simulink model "fault_solution_mod"  (R2018b)
settings: Solver=VariableStepAuto  StartTime=0.0  StopTime=10  RelTol=1e-3
values from neighbouring files (symbols this model uses):
  E = [1;1;0;0]    [fault.m]
  F = A1 - K1*C    [fault.m]
  Fx = [1;1;1;1]    [fault.m]
  Fy = [1;1]    [fault.m]
  H = E/((C*E)'*(C*E)) * (C*E)'    [fault.m]
  K = K1 + F*H    [fault.m]
  TB = T*B    [fault.m]
undefined symbols (not defined in the file or in its folder): A, B, C
settings Model: Creator=jal  LastModifiedBy=Ion Sircu

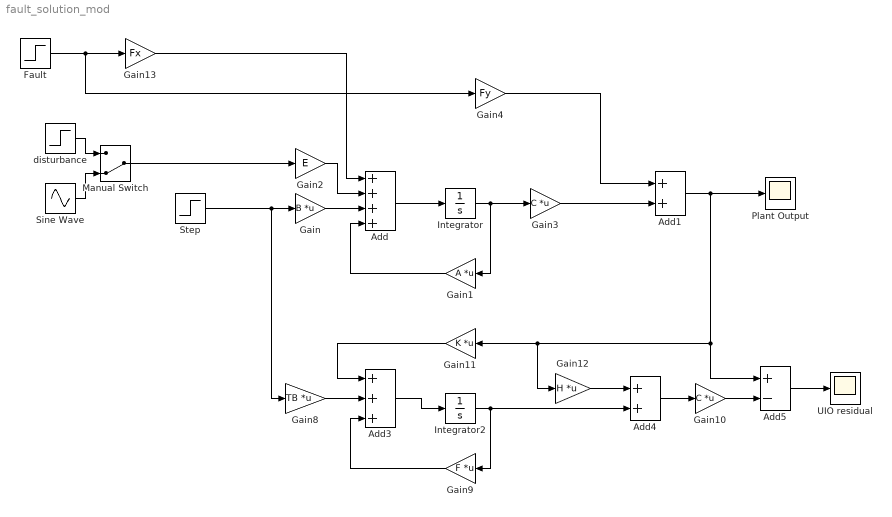
== system fault_solution_mod ==
  Add : Sum  Inputs=++++
  Add1 : Sum
  Add3 : Sum  Inputs=+++
  Add4 : Sum
  Add5 : Sum  Inputs=+-
  Fault : Step  Time=5  After=10  SampleTime=0
  Gain : Gain  Gain=B  Multiplication=Matrix(K*u)
  Gain1 : Gain  Gain=A  Multiplication=Matrix(K*u)
  Gain10 : Gain  Gain=C  Multiplication=Matrix(K*u)
  Gain11 : Gain  Gain=K  Multiplication=Matrix(K*u)
  Gain12 : Gain  Gain=H  Multiplication=Matrix(K*u)
  Gain13 : Gain  Gain=Fx
  Gain2 : Gain  Gain=E
  Gain3 : Gain  Gain=C  Multiplication=Matrix(K*u)
  Gain4 : Gain  Gain=Fy
  Gain8 : Gain  Gain=TB  Multiplication=Matrix(K*u)
  Gain9 : Gain  Gain=F  Multiplication=Matrix(K*u)
  Integrator : Integrator  InitialCondition=[1 1 1 1]
  Integrator2 : Integrator
  Manual Switch : ManualSwitch  CurrentSetting=0
  Plant Output : Scope
  Sine Wave : Sin  SampleTime=0
  Step : Step  SampleTime=0
  UIO residual : Scope
  disturbance : Step  After=10  SampleTime=0
  wires:
  Add/1 -> Integrator/1
  Gain2/1 -> Add/2
  Gain/1 -> Add/3
  Gain1/1 -> Add/4
  Integrator/1 -> Gain1/1, Gain3/1
  Gain3/1 -> Add1/2
  Gain11/1 -> Add3/1
  Add3/1 -> Integrator2/1
  Gain8/1 -> Add3/2
  Gain9/1 -> Add3/3
  Integrator2/1 -> Gain9/1, Add4/2
  Step/1 -> Gain8/1, Gain/1
  Add4/1 -> Gain10/1
  Gain10/1 -> Add5/2
  Add5/1 -> UIO residual/1
  Gain13/1 -> Add/1
  disturbance/1 -> Manual Switch/1
  Manual Switch/1 -> Gain2/1
  Sine Wave/1 -> Manual Switch/2
  Fault/1 -> Gain4/1, Gain13/1
  Gain4/1 -> Add1/1
  Add1/1 -> Plant Output/1, Gain11/1, Gain12/1, Add5/1
  Gain12/1 -> Add4/1
